simulink model "disturbed_kalman"  (R2019b)
settings: Solver=VariableStepAuto  StartTime=0.0  StopTime=10.0  RelTol=1e-3
values from neighbouring files (symbols this model uses):
  A_KF = A_tau + K*C_tau    [matrix_creation.m]
  A_KF_red = A + K(1:n_kf)*C    [matrix_creation.m]
  B_KF = [Bu_tau, -K]    [matrix_creation.m]
  B_KF_red = [Bu, -K(1:n_kf)]    [matrix_creation.m]
  B_simu = [Bu_simu, Bw_simu]    [matrix_creation.m]
  C_KF = eye( n_kf, n_kf )    [matrix_creation.m]
  C_KF_red = eye( n_kf, n_kf)    [matrix_creation.m]
  C_simu_state = eye( n_en, n_en)    [matrix_creation.m]
  D_KF = zeros(n_kf, m_kf)    [matrix_creation.m]
  D_KF_red = zeros(n_kf, m_kf)    [matrix_creation.m]
  D_simu = [Du_simu, Dw_simu]    [matrix_creation.m]
  D_simu_state = zeros(n_en, m_en)    [matrix_creation.m]
  Du = 0.3    [matrix_creation.m]
  tau = 3    [matrix_creation.m]
undefined symbols (not defined in the file or in its folder): A_simu, C_simu
libraries: simulink x3
settings Model: Creator=denniszanutto  LastModifiedBy=denniszanutto

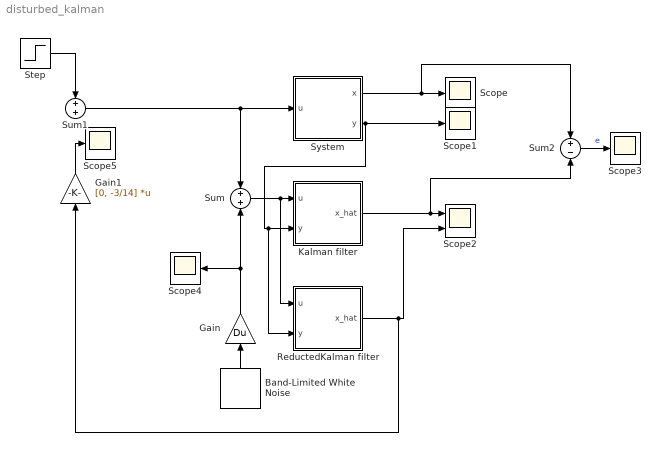
== system disturbed_kalman ==
  Band-Limited White Noise : simulink/Sources/Band-Limited White Noise  Cov=1  Ts=0.1  seed=[23341]
  Gain : Gain  Gain=Du
  Gain1 : Gain  Gain=[0, -3/14]  Multiplication=Matrix(K*u) (u vector)
  Kalman filter : Subsystem
  ReductedKalman filter : Subsystem
  Scope{,1,3..5} (5 alike) : Scope
  Scope2 : Scope  NumInputPorts=2
  Step : Step  SampleTime=0
  Sum : Sum
  Sum1 : Sum
  Sum2 : Sum  Inputs=+-
  System : Subsystem
  wires:
  System/1(x) -> Scope/1, Sum2/1
  System/2("y ") -> Kalman filter/2(y), ReductedKalman filter/2(y), Scope1/1
  Sum1/1 -> Sum/1, System/1(u)
  Sum/1 -> ReductedKalman filter/1(u), Kalman filter/1(u)
  Kalman filter/1(x_hat) -> Sum2/2, Scope2/1
  Step/1 -> Sum1/1
  Sum2/1 -> Scope3/1  "e"
  Band-Limited White Noise/1 -> Gain/1
  Gain/1 -> Sum/2, Scope4/1
  ReductedKalman filter/1(x_hat) -> Gain1/1, Scope2/2
  Gain1/1 -> Scope5/1

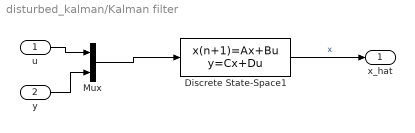
== system disturbed_kalman/Kalman filter ==
  u : Inport
  y : Inport  Port=2
  Discrete State-Space1 : DiscreteStateSpace  A=A_KF  B=B_KF  C=C_KF  D=D_KF  SampleTime=-1
  Mux : Mux  Inputs=2
      settings: DisplayOption=signals
  x_hat : Outport
  wires:
  Discrete State-Space1/1 -> x_hat/1  "x"
  u/1 -> Mux/1
  y/1 -> Mux/2
  Mux/1 -> Discrete State-Space1/1

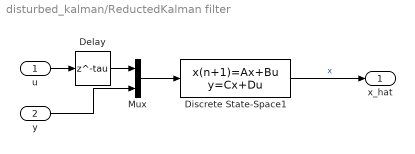
== system disturbed_kalman/ReductedKalman filter ==
  u : Inport
  y : Inport  Port=2
  Delay : Delay  DelayLength=tau
  Discrete State-Space1 : DiscreteStateSpace  A=A_KF_red  B=B_KF_red  C=C_KF_red  D=D_KF_red  SampleTime=-1
  Mux : Mux  Inputs=2
      settings: DisplayOption=signals
  x_hat : Outport
  wires:
  Discrete State-Space1/1 -> x_hat/1  "x"
  y/1 -> Mux/2
  Mux/1 -> Discrete State-Space1/1
  u/1 -> Delay/1
  Delay/1 -> Mux/1

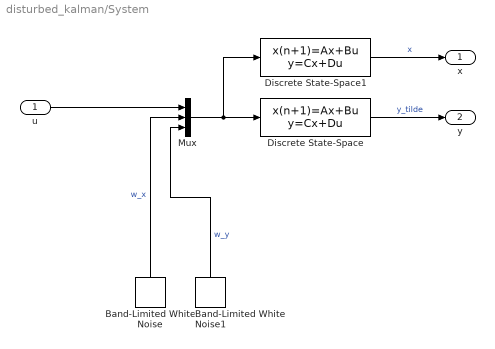
== system disturbed_kalman/System ==
  u : Inport
  Band-Limited White Noise : simulink/Sources/Band-Limited White Noise  Cov=1  Ts=0.1  seed=[23341]
  Band-Limited White Noise1 : simulink/Sources/Band-Limited White Noise  Cov=1  Ts=0.1  seed=[23341]
  Discrete State-Space : DiscreteStateSpace  A=A_simu  B=B_simu  C=C_simu  D=D_simu  SampleTime=-1
  Discrete State-Space1 : DiscreteStateSpace  A=A_simu  B=B_simu  C=C_simu_state  D=D_simu_state  SampleTime=-1
  Mux : Mux  Inputs=3
  x : Outport
  "y " : Outport  Port=2
  wires:
  Discrete State-Space1/1 -> x/1  "x"
  Discrete State-Space/1 -> "y "/1  "y_tilde"
  Mux/1 -> Discrete State-Space1/1, Discrete State-Space/1
  Band-Limited White Noise/1 -> Mux/2  "w_x"
  Band-Limited White Noise1/1 -> Mux/3  "w_y"
  u/1 -> Mux/1
